simulink model "qpsk"  (Simulink 6.4)
settings: Solver=FixedStepDiscrete  StartTime=0.0  StopTime=20  RelTol=1e-3
undefined symbols (not defined in the file or in its folder): get
libraries: commdigbbndpm3 x3, commsink2 x3, commchan3 x1, dspbuff3 x1, commrandsrc2 x1
settings Model: Creator=ALEX  LastModifiedBy=student
settings OptimizationCC: InitFltsAndDblsToZero=off
settings DebuggingCC: SignalResolutionControl=UseLocalSettings  MultiTaskDSMMsg=error  MultiTaskCondExecSysMsg=error
settings GRTTargetCC: TargetFcnLib=ansi_tfl_table_tmw.mat

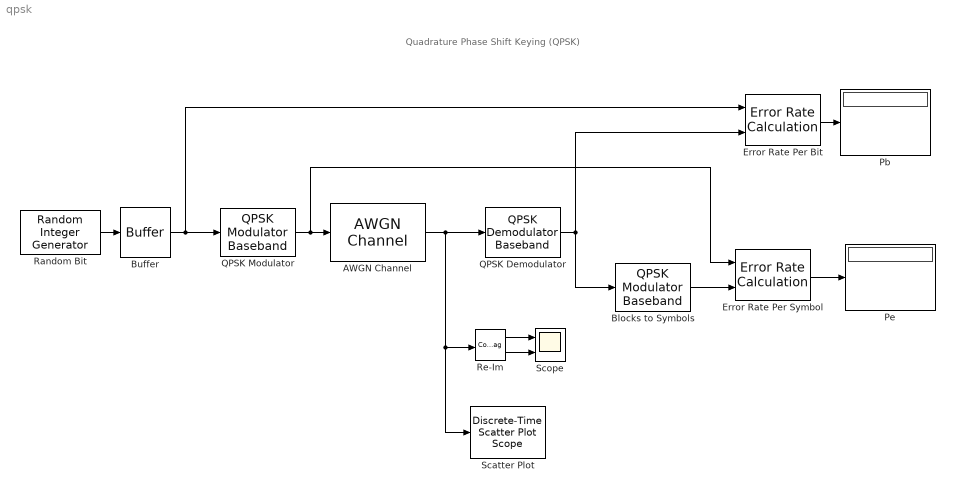
== system qpsk ==
  note: Quadrature Phase Shift Keying (QPSK)
  AWGN Channel : commchan3/AWGN Channel  SystemSampleTime=-1  seed=67  noiseMode="Signal to noise ratio  (Es/No)"  EbNodB=6  EsNodB=100  SNRdB=10  bitsPerSym=2  Ps=1  Tsym=1  variance=0
  Blocks to Symbols : commdigbbndpm3/QPSK Modulator Baseband  SystemSampleTime=-1  InType=Bit  Enc=Gray  Ph=pi/4  outDtype=double  outWordLen=16  outUDDataType=sfix(16)  outFracLenMode=Best precision  outFracLen=15
  Buffer : dspbuff3/Buffer  N=2  V=0  ic=0
  Error Rate Per Bit : commsink2/Error Rate Calculation  N=0  st_delay=0  cp_mode=Entire frame  subframe=[]  PMode=Port  WsName=ErrorVec  RsMode2=off  stop=off  numErr=10  maxBits=100000
  Error Rate Per Symbol : commsink2/Error Rate Calculation  N=0  st_delay=0  cp_mode=Entire frame  subframe=[]  PMode=Port  WsName=ErrorVec  RsMode2=off  stop=off  numErr=10  maxBits=100000
  Pb : Display
  Pe : Display
  QPSK Demodulator : commdigbbndpm3/QPSK Demodulator Baseband  SystemSampleTime=-1  OutType=Bit  Dec=Binary  Ph=pi/4  outDtype1=boolean  outDtype2=double
  QPSK Modulator : commdigbbndpm3/QPSK Modulator Baseband  SystemSampleTime=-1  InType=Bit  Enc=Gray  Ph=pi/4  outDtype=double  outWordLen=16  outUDDataType=sfix(16)  outFracLenMode=Best precision  outFracLen=15
  Random Bit : commrandsrc2/Random Integer Generator  SystemSampleTime=-1  mul=2  seed=37  Ts=0.5  frameBased=off  sampPerFrame=8  orient=on  outDataType=boolean
  Re-Im : ComplexToRealImag
  Scatter Plot : commsink2/Discrete-Time Scatter Plot Scope  Tag=ScatterPlot  SystemSampleTime=-1  sampPerSymb=1  offsetEye=0  numTraces=100  numNewFrames=10  LineMarkers=.  LineColors=b  fading=on  render=on  AxisGrid=on  xMin=-2  xMax=2  yMin=-2  yMax=2  inphaseLabel=In-phase Amplitude  quadratureLabel=Quadrature Amplitude  openScopeAtSimStart=off  FrameNumber=off  FigPos=get(0,'defaultfigureposition');  figTitle=Scatter Plot  numLinesMax=8  block_type_=scatter
  Scope : Scope  NumInputPorts=2
      settings: YMin=-1.2~-1.2  YMax=1.2~1.2
  wires:
  Error Rate Per Bit/1 -> Pb/1
  AWGN Channel/1 -> QPSK Demodulator/1, Scatter Plot/1, Re-Im/1
  QPSK Demodulator/1 -> Error Rate Per Bit/2, Blocks to Symbols/1
  Random Bit/1 -> Buffer/1
  Re-Im/1 -> Scope/1
  Re-Im/2 -> Scope/2
  Buffer/1 -> QPSK Modulator/1, Error Rate Per Bit/1
  Error Rate Per Symbol/1 -> Pe/1
  QPSK Modulator/1 -> AWGN Channel/1, Error Rate Per Symbol/1
  Blocks to Symbols/1 -> Error Rate Per Symbol/2
